simulink model "Astrobee_Simulink_template"  (R2023b)
settings: Solver=FixedStepDiscrete  StartTime=0.0  StopTime=Inf  FixedStep=0.02  RelTol=1e-3  EnableMultiTasking=on
undefined symbols (not defined in the file or in its folder): Header, Wrench
libraries: robotlib x6, simulink x4
settings Model: Creator=The MathWorks, Inc.  LastModifiedBy=Yazan
settings SolverCC: AlgebraicLoopSolver=TrustRegion
settings DataIOCC: LimitDataPoints=on  SaveFormat=Array  ReturnWorkspaceOutputs=off
settings OptimizationCC: ZeroExternalMemoryAtStartup=off  ZeroInternalMemoryAtStartup=off  LifeSpan=Inf  MaxStackSize=64
settings DebuggingCC: SolverPrmCheckMsg=warning  UnconnectedInputMsg=warning  UnconnectedOutputMsg=warning  UnconnectedLineMsg=warning  AllowSymbolicDim=off  SFUnexpectedBacktrackingDiag=warning  SFNoUnconditionalDefaultTransitionDiag=warning  SFExecutionAtInitializationDiag=none  ArithmeticOperatorsInVariantConditions=warning
settings HardwareCC: ProdBitPerPointer=32  ProdBitPerSizeT=32  ProdBitPerPtrDiffT=32  ProdLargestAtomicFloat=None  ProdIntDivRoundTo=Undefined  ProdEndianess=Unspecified  ProdWordSize=32  ProdHWDeviceType=Generic->Unspecified (assume 32-bit Generic)  TargetHWDeviceType=Generic->Unspecified (assume 32-bit Generic)  UseEmbeddedCoderFeatures=off
settings ModelReferenceCC: EnableRefExpFcnMdlSchedulingChecks=on  PropagateSignalLabelsOutOfModel=off
settings SFSimCC: SimUseLocalCustomCode=off  CustomCodeUndefinedFunction=UseInterfaceOnly  SimTargetLang=C++
settings RTWCC: Description=Embedded Coder  SystemTargetFile=ert.tlc  HardwareBoard=Robot Operating System (ROS)  TemplateMakefile=ert_default_tmf  RTWUseLocalCustomCode=off  Toolchain=Catkin  TargetLang=C++
settings CodeAppCC: StateflowObjectComments=on
settings ERTTargetCC: MultiwordLength=2048  ERTCustomFileBanners=off  CodeInterfacePackaging=C++ class  SupportContinuousTime=on  SupportNonInlinedSFcns=on  RemoveResetFunc=off  SupportVariableSizeSignals=on  ModelStepFunctionPrototypeControlCompliant=off  RootIOFormat=Structure reference  ConvertIfToSwitch=off  SuppressUnreachableDefaultCases=off
settings ConfigComp: CovMetricSettings=dw  CovSaveCumulativeToWorkspaceVar=on  CovSaveSingleToWorkspaceVar=on  CovExternalEMLEnable=off  CovSFcnEnable=off

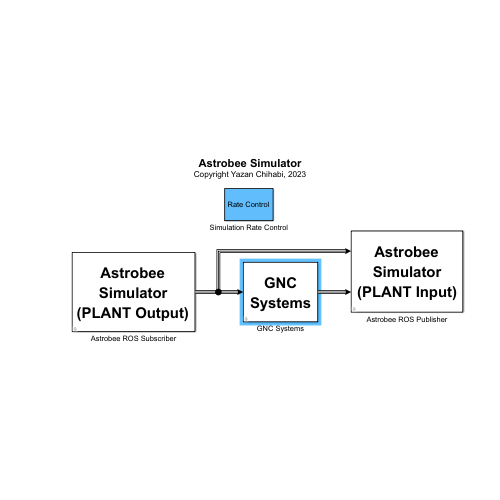
[thumbnail: Simulink's stored preview of the top-level diagram]
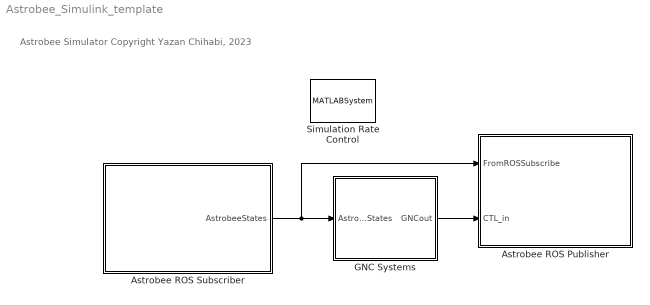
== system Astrobee_Simulink_template ==
  note: Astrobee Simulator
      | Copyright Yazan Chihabi, 2023
  Astrobee ROS Publisher : Subsystem
      mask Display: disp(['{\bf\fontsize{20}Astrobee}' newline newline '{\bf\fontsize{20}Simulator}' newline newline '{\bf\fontsize{20}(PLANT Input)}'], 'texmode','on');
  Astrobee ROS Subscriber : Subsystem
      mask Display: disp(['{\bf\fontsize{20}Astrobee}' newline newline '{\bf\fontsize{20}Simulator}' newline newline '{\bf\fontsize{20}(PLANT Output)}'], 'texmode','on');
  GNC Systems : Subsystem
      mask Display: disp(['{\bf\fontsize{20}GNC}' newline newline '{\bf\fontsize{20}Systems}'], 'texmode','on');
  Simulation Rate Control : MATLABSystem  System=AstrobeeSimulationRateControl  SampleTime=0.02
      mask Type: AstrobeeSimulationRateControl
      mask Display: disp('Rate Control');
  wires:
  Astrobee ROS Subscriber/1(AstrobeeStates) -> Astrobee ROS Publisher/1(FromROSSubscribe), GNC Systems/1(AstrobeeStates)
  GNC Systems/1(GNCout) -> Astrobee ROS Publisher/2(CTL_in)

== system Astrobee_Simulink_template/Astrobee ROS Publisher ==
  FromROSSubscribe : Inport
  CTL_in : Inport  Port=2
  Bus Selector : BusSelector  OutputSignals=HoneyStates.IsNew,BumbleStates.IsNew
  Command Thrust/Torque Publisher (Bumble) : Subsystem
  Command Thrust/Torque Publisher (Honey) : Subsystem
  wires:
  CTL_in/1 -> Command Thrust/Torque Publisher (Honey)/1(CTL_in), Command Thrust/Torque Publisher (Bumble)/1(CTL_in)
  Bus Selector/1 -> Command Thrust/Torque Publisher (Honey)/Enable  "<IsNew>"
  FromROSSubscribe/1 -> Bus Selector/1
  Bus Selector/2 -> Command Thrust/Torque Publisher (Bumble)/Enable  "<IsNew>"

== system Astrobee_Simulink_template/Astrobee ROS Subscriber ==
  Bus Creator : BusCreator  Inputs=2
  ROS Subscriber - Bumble : Subsystem
  ROS Subscriber - Honey : Subsystem
  AstrobeeStates : Outport
  wires:
  ROS Subscriber - Bumble/1(BumbleStates) -> Bus Creator/2
  ROS Subscriber - Honey/1(HoneyStates) -> Bus Creator/1
  Bus Creator/1 -> AstrobeeStates/1

== system Astrobee_Simulink_template/GNC Systems ==
  AstrobeeStates : Inport
  Bumble : Subsystem
      mask Display: disp(['{\bf\fontsize{20}Bumble}' newline newline '{\bf\fontsize{20}GNC}'], 'texmode','on');
  Bus Creator : BusCreator  Inputs=2
  Honey : Subsystem
      mask Display: disp(['{\bf\fontsize{20}Honey}' newline newline '{\bf\fontsize{20}GNC}'], 'texmode','on');
  GNCout : Outport
  wires:
  AstrobeeStates/1 -> Bumble/1(AstrobeeStates), Honey/1(AstrobeeStates)
  Bumble/1(Out1) -> Bus Creator/2
  Honey/1(Out1) -> Bus Creator/1
  Bus Creator/1 -> GNCout/1  "GNCout"

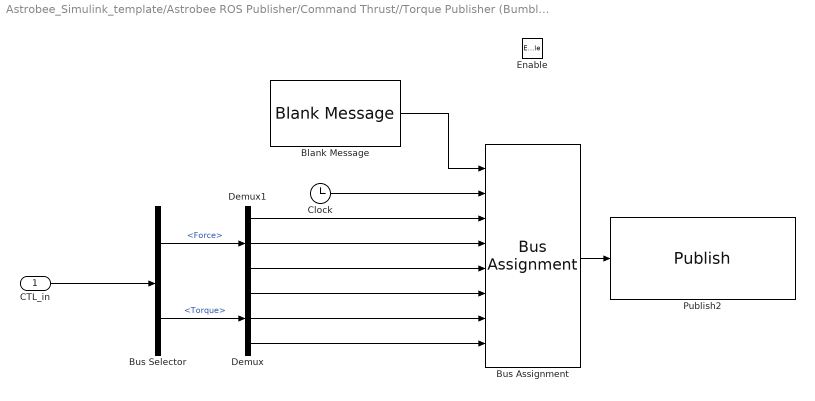
== system Astrobee_Simulink_template/Astrobee ROS Publisher/Command Thrust//Torque Publisher (Bumble) ==
  CTL_in : Inport
  Enable : EnablePort
  Blank Message : robotlib/Blank Message  messageClass=Message  entityType=ff_msgs/FamCommand  messageType=ff_msgs/FamCommand  SampleTime=inf  legacyBusStruct=off
  Bus Assignment : BusAssignment  AssignedSignals=Header.Stamp.Sec,Wrench.Force.X,Wrench.Force.Y,Wrench.Force.Z,Wrench.Torque.X,Wrench.Torque.Y,Wrench.Torque.Z
  Bus Selector : BusSelector  OutputSignals=BumbleCTL.Force,BumbleCTL.Torque
  Clock : Clock
  Demux : Demux  Outputs=3
  Demux1 : Demux  Outputs=3
  Publish2 : robotlib/Publish  topicSource=Select from ROS network  topic=/bumble/gnc/ctl/command  messageType=ff_msgs/FamCommand  legacyBusStruct=off  messageQueueLength=105
  wires:
  CTL_in/1 -> Bus Selector/1
  Bus Selector/1 -> Demux1/1  "<Force>"
  Bus Selector/2 -> Demux/1  "<Torque>"
  Demux1/1 -> Bus Assignment/3
  Demux1/2 -> Bus Assignment/4
  Demux1/3 -> Bus Assignment/5
  Demux/3 -> Bus Assignment/8
  Demux/2 -> Bus Assignment/7
  Demux/1 -> Bus Assignment/6
  Clock/1 -> Bus Assignment/2
  Bus Assignment/1 -> Publish2/1
  Blank Message/1 -> Bus Assignment/1

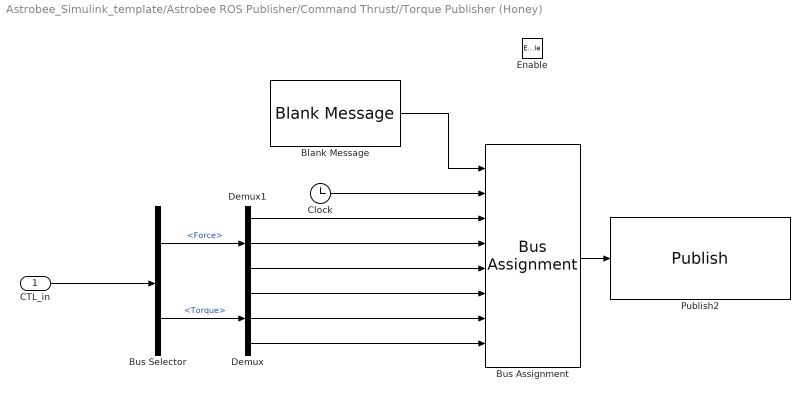
== system Astrobee_Simulink_template/Astrobee ROS Publisher/Command Thrust//Torque Publisher (Honey) ==
  CTL_in : Inport
  Enable : EnablePort
  Blank Message : robotlib/Blank Message  messageClass=Message  entityType=ff_msgs/FamCommand  messageType=ff_msgs/FamCommand  SampleTime=inf  legacyBusStruct=off
  Bus Assignment : BusAssignment  AssignedSignals=Header.Stamp.Sec,Wrench.Force.X,Wrench.Force.Y,Wrench.Force.Z,Wrench.Torque.X,Wrench.Torque.Y,Wrench.Torque.Z
  Bus Selector : BusSelector  OutputSignals=HoneyCTL.Force,HoneyCTL.Torque
  Clock : Clock
  Demux : Demux  Outputs=3
  Demux1 : Demux  Outputs=3
  Publish2 : robotlib/Publish  topicSource=Select from ROS network  topic=/honey/gnc/ctl/command  messageType=ff_msgs/FamCommand  legacyBusStruct=off  messageQueueLength=105
  wires:
  Blank Message/1 -> Bus Assignment/1
  Bus Assignment/1 -> Publish2/1
  Clock/1 -> Bus Assignment/2
  Demux/1 -> Bus Assignment/6
  Demux/2 -> Bus Assignment/7
  Demux/3 -> Bus Assignment/8
  Demux1/3 -> Bus Assignment/5
  Demux1/2 -> Bus Assignment/4
  Demux1/1 -> Bus Assignment/3
  Bus Selector/2 -> Demux/1  "<Torque>"
  Bus Selector/1 -> Demux1/1  "<Force>"
  CTL_in/1 -> Bus Selector/1

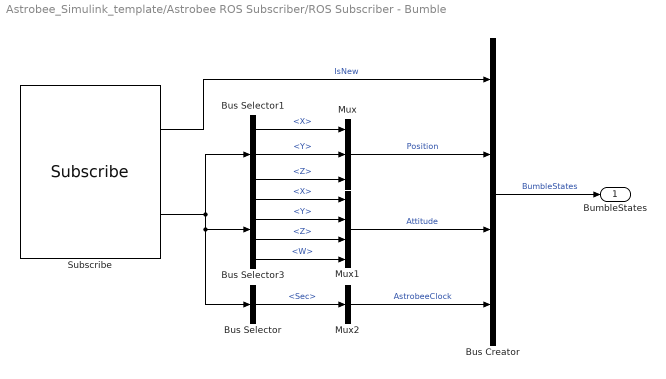
== system Astrobee_Simulink_template/Astrobee ROS Subscriber/ROS Subscriber - Bumble ==
  Bus Creator : BusCreator  Inputs=4
  Bus Selector : BusSelector  OutputSignals=Header.Stamp.Sec
  Bus Selector1 : BusSelector  OutputSignals=Pose.Position.X,Pose.Position.Y,Pose.Position.Z
  Bus Selector3 : BusSelector  OutputSignals=Pose.Orientation.X,Pose.Orientation.Y,Pose.Orientation.Z,Pose.Orientation.W
  Mux : Mux  Inputs=3
  Mux1 : Mux
  Mux2 : Mux  Inputs=1
  Subscribe : robotlib/Subscribe  topicSource=Select from ROS network  topic=/bumble/gnc/ekf  messageType=ff_msgs/EkfState  SampleTime=-1  legacyBusStruct=off  messageQueueLength=51
  BumbleStates : Outport
  wires:
  Bus Creator/1 -> BumbleStates/1  "BumbleStates"
  Bus Selector/1 -> Mux2/1  "<Sec>"
  Bus Selector1/1 -> Mux/1  "<X>"
  Bus Selector1/3 -> Mux/3  "<Z>"
  Bus Selector1/2 -> Mux/2  "<Y>"
  Mux2/1 -> Bus Creator/4  "AstrobeeClock"
  Mux1/1 -> Bus Creator/3  "Attitude"
  Bus Selector3/2 -> Mux1/2  "<Y>"
  Mux/1 -> Bus Creator/2  "Position"
  Bus Selector3/1 -> Mux1/1  "<X>"
  Bus Selector3/3 -> Mux1/3  "<Z>"
  Subscribe/1 -> Bus Creator/1  "IsNew"
  Bus Selector3/4 -> Mux1/4  "<W>"
  Subscribe/2 -> Bus Selector/1, Bus Selector3/1, Bus Selector1/1

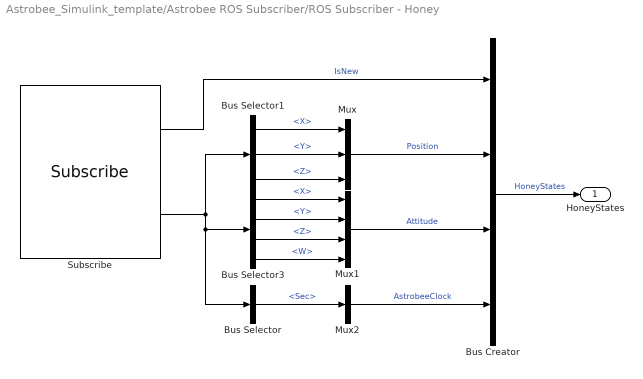
== system Astrobee_Simulink_template/Astrobee ROS Subscriber/ROS Subscriber - Honey ==
  Bus Creator : BusCreator  Inputs=4
  Bus Selector : BusSelector  OutputSignals=Header.Stamp.Sec
  Bus Selector1 : BusSelector  OutputSignals=Pose.Position.X,Pose.Position.Y,Pose.Position.Z
  Bus Selector3 : BusSelector  OutputSignals=Pose.Orientation.X,Pose.Orientation.Y,Pose.Orientation.Z,Pose.Orientation.W
  Mux : Mux  Inputs=3
  Mux1 : Mux
  Mux2 : Mux  Inputs=1
  Subscribe : robotlib/Subscribe  topicSource=Select from ROS network  topic=/honey/gnc/ekf  messageType=ff_msgs/EkfState  SampleTime=-1  legacyBusStruct=off  messageQueueLength=51
  HoneyStates : Outport
  wires:
  Subscribe/2 -> Bus Selector1/1, Bus Selector3/1, Bus Selector/1
  Bus Selector3/4 -> Mux1/4  "<W>"
  Subscribe/1 -> Bus Creator/1  "IsNew"
  Bus Selector3/3 -> Mux1/3  "<Z>"
  Bus Selector3/1 -> Mux1/1  "<X>"
  Mux/1 -> Bus Creator/2  "Position"
  Bus Selector3/2 -> Mux1/2  "<Y>"
  Mux1/1 -> Bus Creator/3  "Attitude"
  Mux2/1 -> Bus Creator/4  "AstrobeeClock"
  Bus Selector1/2 -> Mux/2  "<Y>"
  Bus Selector1/3 -> Mux/3  "<Z>"
  Bus Selector1/1 -> Mux/1  "<X>"
  Bus Selector/1 -> Mux2/1  "<Sec>"
  Bus Creator/1 -> HoneyStates/1  "HoneyStates"

== system Astrobee_Simulink_template/GNC Systems/Bumble ==
  AstrobeeStates : Inport
  Bus Selector : BusSelector  OutputSignals=BumbleStates.IsNew
  Simple Controller : Subsystem
  Out1 : Outport
  wires:
  Simple Controller/1(CTL_out) -> Out1/1  "BumbleCTL"
  AstrobeeStates/1 -> Simple Controller/1(States), Bus Selector/1
  Bus Selector/1 -> Simple Controller/Enable  "<IsNew>"

== system Astrobee_Simulink_template/GNC Systems/Honey ==
  AstrobeeStates : Inport
  Bus Selector : BusSelector  OutputSignals=HoneyStates.IsNew
  Simple Controller : Subsystem
  Out1 : Outport
  wires:
  Bus Selector/1 -> Simple Controller/Enable  "<IsNew>"
  AstrobeeStates/1 -> Bus Selector/1, Simple Controller/1(States)
  Simple Controller/1(CTL_out) -> Out1/1  "HoneyCTL"

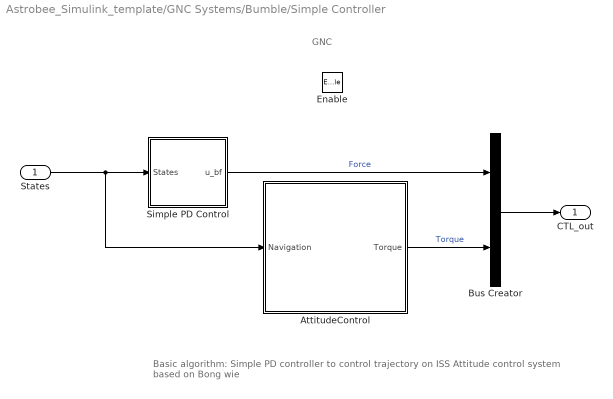
== system Astrobee_Simulink_template/GNC Systems/Bumble/Simple Controller ==
  note: Basic algorithm:
      | Simple PD controller to control trajectory on ISS
      | Attitude control system based on Bong wie
  note: GNC
  States : Inport
  Enable : EnablePort
  AttitudeControl : Subsystem
      mask Display: disp(['{\bf\fontsize{20}Attitude}' newline newline '{\bf\fontsize{20}Control}' newline newline '{\bf\fontsize{20}System}'], 'texmode','on');
  Bus Creator : BusCreator  Inputs=2
  Simple PD Control : Subsystem
  CTL_out : Outport
  wires:
  Bus Creator/1 -> CTL_out/1
  Simple PD Control/1(u_bf) -> Bus Creator/1  "Force"
  AttitudeControl/1(Torque) -> Bus Creator/2  "Torque"
  States/1 -> Simple PD Control/1(States), AttitudeControl/1(Navigation)

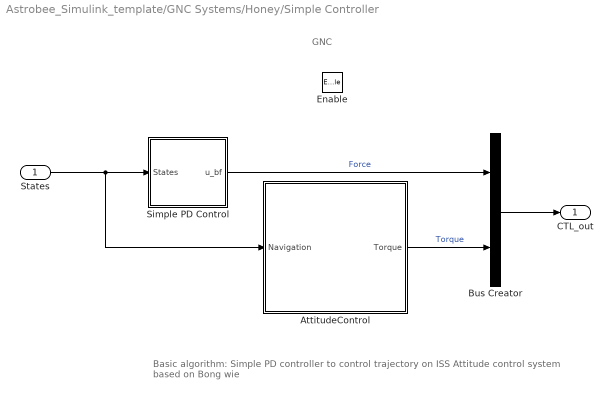
== system Astrobee_Simulink_template/GNC Systems/Honey/Simple Controller ==
  note: GNC
  note: Basic algorithm:
      | Simple PD controller to control trajectory on ISS
      | Attitude control system based on Bong wie
  States : Inport
  Enable : EnablePort
  AttitudeControl : Subsystem
      mask Display: disp(['{\bf\fontsize{20}Attitude}' newline newline '{\bf\fontsize{20}Control}' newline newline '{\bf\fontsize{20}System}'], 'texmode','on');
  Bus Creator : BusCreator  Inputs=2
  Simple PD Control : Subsystem
  CTL_out : Outport
  wires:
  States/1 -> AttitudeControl/1(Navigation), Simple PD Control/1(States)
  AttitudeControl/1(Torque) -> Bus Creator/2  "Torque"
  Simple PD Control/1(u_bf) -> Bus Creator/1  "Force"
  Bus Creator/1 -> CTL_out/1

== system Astrobee_Simulink_template/GNC Systems/Bumble/Simple Controller/AttitudeControl ==
  Navigation : Inport
  AttitudeController : Subsystem
  Constant : Constant  Value=[0;0;0;1]
  QuaternionError : Subsystem
  Torque : Outport  VectorParamsAs1DForOutWhenUnconnected=off
  wires:
  AttitudeController/1(Control) -> Torque/1
  QuaternionError/1(q_error) -> AttitudeController/1(Error)
  Constant/1 -> QuaternionError/1(qd)
  Navigation/1 -> AttitudeController/2(Nav), QuaternionError/2(" Navigation")

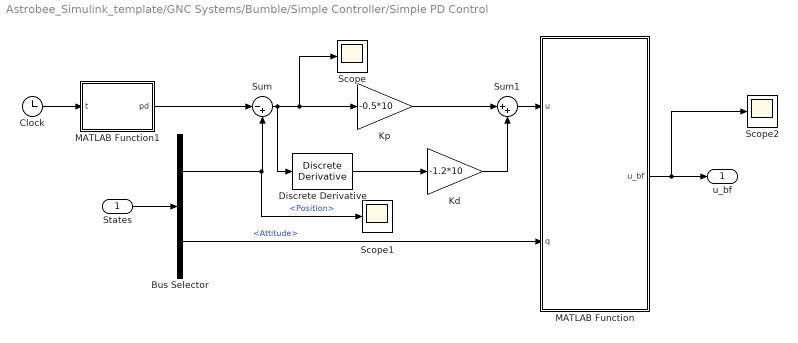
== system Astrobee_Simulink_template/GNC Systems/Bumble/Simple Controller/Simple PD Control ==
  States : Inport
  Bus Selector : BusSelector  OutputSignals=BumbleStates.Position,BumbleStates.Attitude
  Clock : Clock
  Discrete Derivative : simulink/Discrete/Discrete Derivative  gainval=1.0  ICPrevScaledInput=0.0  OutMin=[]  OutMax=[]  OutDataType=fixdt(1, 16)  OutScaling=2^-10  DoSatur=off
  Kd : Gain  Gain=-1.2*10
  Kp : Gain  Gain=-0.5*10
  MATLAB Function : MATLAB Function  TreatAsAtomicUnit=on
  MATLAB Function1 : MATLAB Function  TreatAsAtomicUnit=on
  Scope : Scope
  Scope1 : Scope
  Scope2 : Scope
  Sum : Sum  Inputs=|-+
  Sum1 : Sum  Inputs=|++
  u_bf : Outport
  wires:
  Clock/1 -> MATLAB Function1/1(t)
  Kd/1 -> Sum1/2
  Sum1/1 -> MATLAB Function/1(u)
  MATLAB Function/1(u_bf) -> u_bf/1, Scope2/1
  Bus Selector/2 -> MATLAB Function/2(q)  "<Attitude>"
  Bus Selector/1 -> Sum/2, Scope1/1  "<Position>"
  Kp/1 -> Sum1/1
  States/1 -> Bus Selector/1
  Sum/1 -> Kp/1, Scope/1, Discrete Derivative/1
  MATLAB Function1/1(pd) -> Sum/1
  Discrete Derivative/1 -> Kd/1

== system Astrobee_Simulink_template/GNC Systems/Honey/Simple Controller/AttitudeControl ==
  Navigation : Inport
  AttitudeController : Subsystem
  Constant : Constant  Value=[0;0;sin(-pi/4);cos(-pi/4)]
  QuaternionError : Subsystem
  Torque : Outport  VectorParamsAs1DForOutWhenUnconnected=off
  wires:
  Navigation/1 -> QuaternionError/2(" Navigation"), AttitudeController/2(Nav)
  Constant/1 -> QuaternionError/1(qd)
  QuaternionError/1(q_error) -> AttitudeController/1(Error)
  AttitudeController/1(Control) -> Torque/1

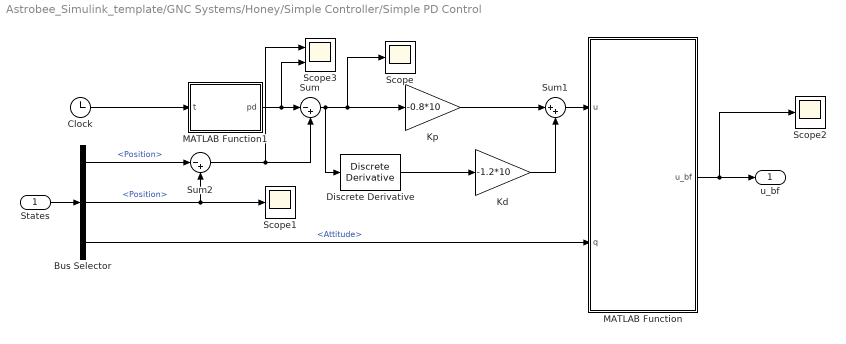
== system Astrobee_Simulink_template/GNC Systems/Honey/Simple Controller/Simple PD Control ==
  States : Inport
  Bus Selector : BusSelector  OutputSignals=BumbleStates.Position,HoneyStates.Position,HoneyStates.Attitude
  Clock : Clock
  Discrete Derivative : simulink/Discrete/Discrete Derivative  gainval=1.0  ICPrevScaledInput=0.0  OutMin=[]  OutMax=[]  OutDataType=fixdt(1, 16)  OutScaling=2^-10  DoSatur=off
  Kd : Gain  Gain=-1.2*10
  Kp : Gain  Gain=-0.8*10
  MATLAB Function : MATLAB Function  TreatAsAtomicUnit=on
  MATLAB Function1 : MATLAB Function  TreatAsAtomicUnit=on
  Scope : Scope
  Scope1 : Scope
  Scope2 : Scope
  Scope3 : Scope  NumInputPorts=2
  Sum : Sum  Inputs=|-+
  Sum1 : Sum  Inputs=|++
  Sum2 : Sum  Inputs=|-+
  u_bf : Outport
  wires:
  Discrete Derivative/1 -> Kd/1
  MATLAB Function1/1(pd) -> Scope3/2, Sum/1
  Sum/1 -> Discrete Derivative/1, Scope/1, Kp/1
  States/1 -> Bus Selector/1
  Kp/1 -> Sum1/1
  Bus Selector/2 -> Scope1/1, Sum2/2  "<Position>"
  Bus Selector/3 -> MATLAB Function/2(q)  "<Attitude>"
  MATLAB Function/1(u_bf) -> Scope2/1, u_bf/1
  Sum1/1 -> MATLAB Function/1(u)
  Kd/1 -> Sum1/2
  Clock/1 -> MATLAB Function1/1(t)
  Bus Selector/1 -> Sum2/1  "<Position>"
  Sum2/1 -> Scope3/1, Sum/2

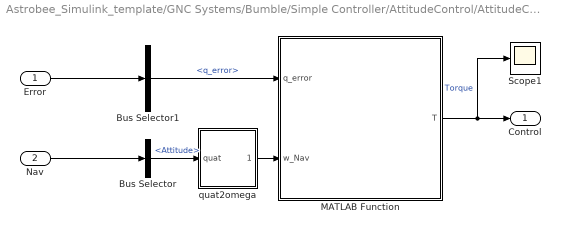
== system Astrobee_Simulink_template/GNC Systems/Bumble/Simple Controller/AttitudeControl/AttitudeController ==
  Error : Inport
  Nav : Inport  Port=2
  Bus Selector : BusSelector  OutputSignals=BumbleStates.Attitude
  Bus Selector1 : BusSelector  OutputSignals=q_error
  MATLAB Function : MATLAB Function  TreatAsAtomicUnit=on
  Scope1 : Scope
  quat2omega : Subsystem
  Control : Outport
  wires:
  Nav/1 -> Bus Selector/1
  Bus Selector/1 -> quat2omega/1(quat)  "<Attitude>"
  quat2omega/1(omega) -> MATLAB Function/2(w_Nav)
  Error/1 -> Bus Selector1/1
  MATLAB Function/1(T) -> Control/1, Scope1/1  "Torque"
  Bus Selector1/1 -> MATLAB Function/1(q_error)  "<q_error>"

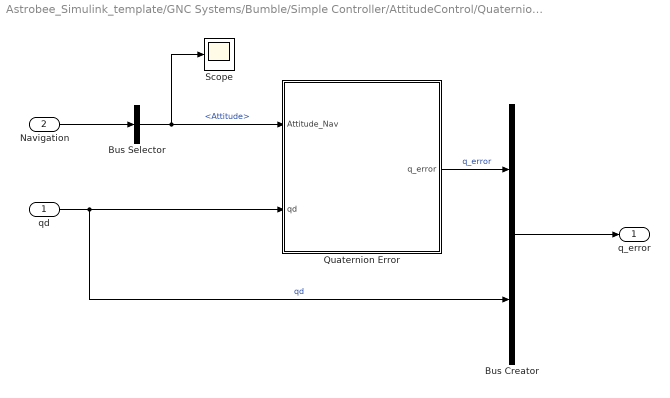
== system Astrobee_Simulink_template/GNC Systems/Bumble/Simple Controller/AttitudeControl/QuaternionError ==
  qd : Inport
  " Navigation" : Inport  Port=2
  Bus Creator : BusCreator  Inputs=2
  Bus Selector : BusSelector  OutputSignals=BumbleStates.Attitude
  Quaternion Error : MATLAB Function  TreatAsAtomicUnit=on
  Scope : Scope
  q_error : Outport  VectorParamsAs1DForOutWhenUnconnected=off
  wires:
  qd/1 -> Quaternion Error/2(qd), Bus Creator/2  "qd"
  Bus Creator/1 -> q_error/1
  Bus Selector/1 -> Scope/1, Quaternion Error/1(Attitude_Nav)  "<Attitude>"
  Quaternion Error/1(q_error) -> Bus Creator/1  "q_error"
  " Navigation"/1 -> Bus Selector/1

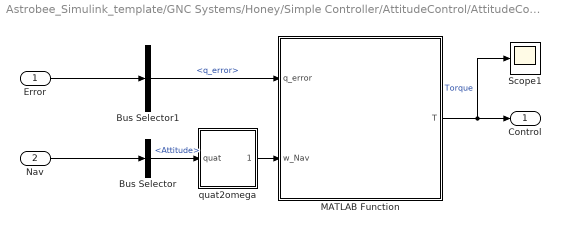
== system Astrobee_Simulink_template/GNC Systems/Honey/Simple Controller/AttitudeControl/AttitudeController ==
  Error : Inport
  Nav : Inport  Port=2
  Bus Selector : BusSelector  OutputSignals=HoneyStates.Attitude
  Bus Selector1 : BusSelector  OutputSignals=q_error
  MATLAB Function : MATLAB Function  TreatAsAtomicUnit=on
  Scope1 : Scope
  quat2omega : Subsystem
  Control : Outport
  wires:
  Bus Selector1/1 -> MATLAB Function/1(q_error)  "<q_error>"
  MATLAB Function/1(T) -> Scope1/1, Control/1  "Torque"
  Error/1 -> Bus Selector1/1
  quat2omega/1(omega) -> MATLAB Function/2(w_Nav)
  Bus Selector/1 -> quat2omega/1(quat)  "<Attitude>"
  Nav/1 -> Bus Selector/1

== system Astrobee_Simulink_template/GNC Systems/Honey/Simple Controller/AttitudeControl/QuaternionError ==
  qd : Inport
  " Navigation" : Inport  Port=2
  Bus Creator : BusCreator  Inputs=2
  Bus Selector : BusSelector  OutputSignals=HoneyStates.Attitude
  Quaternion Error : MATLAB Function  TreatAsAtomicUnit=on
  q_error : Outport  VectorParamsAs1DForOutWhenUnconnected=off
  wires:
  " Navigation"/1 -> Bus Selector/1
  Quaternion Error/1(q_error) -> Bus Creator/1  "q_error"
  Bus Selector/1 -> Quaternion Error/1(Attitude_Nav)  "<Attitude>"
  Bus Creator/1 -> q_error/1
  qd/1 -> Bus Creator/2, Quaternion Error/2(qd)  "qd"

== system Astrobee_Simulink_template/GNC Systems/Bumble/Simple Controller/AttitudeControl/AttitudeController/quat2omega ==
  quat : Inport
  Conversion : MATLAB Function  TreatAsAtomicUnit=on
  Discrete Derivative : simulink/Discrete/Discrete Derivative  gainval=1.0  ICPrevScaledInput=0.0  OutMin=[]  OutMax=[]  OutDataType=fixdt(1, 16)  OutScaling=2^-10  DoSatur=off
  MATLAB Function1 : MATLAB Function  TreatAsAtomicUnit=on
  omega : Outport
  wires:
  quat/1 -> Conversion/1(q)
  MATLAB Function1/1(omega) -> omega/1
  Discrete Derivative/1 -> MATLAB Function1/1(Angle_rate)
  Conversion/1(eul) -> Discrete Derivative/1, MATLAB Function1/2(angle)

== system Astrobee_Simulink_template/GNC Systems/Honey/Simple Controller/AttitudeControl/AttitudeController/quat2omega ==
  quat : Inport
  Conversion : MATLAB Function  TreatAsAtomicUnit=on
  Discrete Derivative : simulink/Discrete/Discrete Derivative  gainval=1.0  ICPrevScaledInput=0.0  OutMin=[]  OutMax=[]  OutDataType=fixdt(1, 16)  OutScaling=2^-10  DoSatur=off
  MATLAB Function1 : MATLAB Function  TreatAsAtomicUnit=on
  omega : Outport
  wires:
  Conversion/1(eul) -> MATLAB Function1/2(angle), Discrete Derivative/1
  Discrete Derivative/1 -> MATLAB Function1/1(Angle_rate)
  MATLAB Function1/1(omega) -> omega/1
  quat/1 -> Conversion/1(q)

== matlab function Astrobee_Simulink_template/GNC Systems/Honey/Simple Controller/AttitudeControl/AttitudeController/MATLAB Function ==
  data: q_error input; T output; w_Nav input
function T  = AttitudeController(q_error,w_Nav)

inertiaMatrix = [0.1422,0,0;
    0,0.1422,0;
    0,0,0.1422];
%% ATTITUDE CONTROL %%
%{   
    Run a quaternion-based PD-like attitude controller that minimizes
    the axis error. If q1_error, q2_error, and q3_error are zero, then
    q4_error must be 1 and therefore there is zero error. So, we must
    drive q1_error, q2_error, and q3_error to zero. The sign of 
    q4_error is used to guide the direction.
    
    Controller adapted from: https://arc.aiaa.org/doi/abs/10.2514/3.19988?journalCode=jgcd
    Dr. Bong Wie Attitude Controller
    Inputs: 
        - quaternion_error_in_servicer_body_frame (4 components, the first 3 are the axis components and the 4th is the angle component)
        - angular_rate_error_in_servicer_body_frame (3 angular rate errors in rad/s in the body-fixed reference frame)
%}

% T = (sign(q_error(4))+(q_error(4) == 0))*Kp_Attitude*q_error(1:3) + Kd_Attitude*w_error;

% T = [0;0;0];
%% Different version of Dr. Bong Wie Attitude Controller
%{   
    Quarternion feedback regulator for spacecraft eigenaxis rotations
    B. Wie, H. Weiss and A. Arapostathis https://doi.org/10.2514/3.20418
%}
    q=q_error(1:3); %error quaternions
    T = (-6*inertiaMatrix*q)+(-12*inertiaMatrix*w_Nav)-(cross(w_Nav,inertiaMatrix*(w_Nav)));
end

== matlab function Astrobee_Simulink_template/GNC Systems/Honey/Simple Controller/AttitudeControl/AttitudeController/quat2omega/Conversion ==
  data: eul output; q input
function eul = quat2eul(q)
%#codegen

% Convert the quaternion to euler angles

C = quat2rot(q);

roll = atan2(C(2,3),C(3,3));
pitch = -asin(C(1,3));
yaw = atan2(C(1,2),C(1,1));

eul = [roll;pitch;yaw];
end

== matlab function Astrobee_Simulink_template/GNC Systems/Honey/Simple Controller/AttitudeControl/QuaternionError/Quaternion Error ==
  data: Attitude_Nav input; q_error output size=4; qd input
function q_error  = q_err_calc(Attitude_Nav,qd)


%% Quaternion Error
q_Nav = Attitude_Nav(1:4);
q_Nav = NormalizeQuaternion(q_Nav);

qm = [ qd(4), qd(3),-qd(2),-qd(1);
      -qd(3), qd(4), qd(1),-qd(2);
       qd(2),-qd(1), qd(4),-qd(3);
       qd(1), qd(2), qd(3), qd(4)];
   
q_error = (qm * q_Nav);

q_error = NormalizeQuaternion(q_error); % normalizing and ensuring q(4) is positive

if isnan(q_error)
    q_error = [0;0;0;0];
end


end

== matlab function Astrobee_Simulink_template/GNC Systems/Bumble/Simple Controller/AttitudeControl/AttitudeController/MATLAB Function ==
  data: q_error input; T output; w_Nav input
function T  = AttitudeController(q_error,w_Nav)

inertiaMatrix = [0.1422,0,0;
    0,0.1422,0;
    0,0,0.1422];
%% ATTITUDE CONTROL %%
%{   
    Run a quaternion-based PD-like attitude controller that minimizes
    the axis error. If q1_error, q2_error, and q3_error are zero, then
    q4_error must be 1 and therefore there is zero error. So, we must
    drive q1_error, q2_error, and q3_error to zero. The sign of 
    q4_error is used to guide the direction.
    
    Controller adapted from: https://arc.aiaa.org/doi/abs/10.2514/3.19988?journalCode=jgcd
    Dr. Bong Wie Attitude Controller
    Inputs: 
        - quaternion_error_in_servicer_body_frame (4 components, the first 3 are the axis components and the 4th is the angle component)
        - angular_rate_error_in_servicer_body_frame (3 angular rate errors in rad/s in the body-fixed reference frame)
%}

% T = (sign(q_error(4))+(q_error(4) == 0))*Kp_Attitude*q_error(1:3) + Kd_Attitude*w_error;

% T = [0;0;0];
%% Different version of Dr. Bong Wie Attitude Controller
%{   
    Quarternion feedback regulator for spacecraft eigenaxis rotations
    B. Wie, H. Weiss and A. Arapostathis https://doi.org/10.2514/3.20418
%}
    q=q_error(1:3); %error quaternions
    T = (-6*inertiaMatrix*q)+(-12*inertiaMatrix*w_Nav)-(cross(w_Nav,inertiaMatrix*(w_Nav)));
end

== matlab function Astrobee_Simulink_template/GNC Systems/Bumble/Simple Controller/AttitudeControl/AttitudeController/quat2omega/Conversion ==
  data: eul output; q input
function eul = quat2eul(q)
%#codegen

% Convert the quaternion to euler angles

C = quat2rot(q);

roll = atan2(C(2,3),C(3,3));
pitch = -asin(C(1,3));
yaw = atan2(C(1,2),C(1,1));

eul = [roll;pitch;yaw];
end

== matlab function Astrobee_Simulink_template/GNC Systems/Honey/Simple Controller/AttitudeControl/AttitudeController/quat2omega/MATLAB Function1 ==
  data: Angle_rate input; omega output; angle input
function omega = EulerRates2Omega(Angle_rate,angle)

roll = angle(1);
roll_dot = Angle_rate(1);
pitch = angle(2);
pitch_dot = Angle_rate(2);
yaw = angle(3);
yaw_dot = Angle_rate(3);

Phi = [1 0 -sin(pitch);
    0 cos(roll) -sin(roll);
    0 sin(roll)/cos(pitch) cos(roll)/cos(pitch)];

omega = Phi*[roll_dot;pitch_dot;yaw_dot];

end

== matlab function Astrobee_Simulink_template/GNC Systems/Bumble/Simple Controller/AttitudeControl/AttitudeController/quat2omega/MATLAB Function1 ==
  data: Angle_rate input; omega output; angle input
function omega = EulerRates2Omega(Angle_rate,angle)

roll = angle(1);
roll_dot = Angle_rate(1);
pitch = angle(2);
pitch_dot = Angle_rate(2);
yaw = angle(3);
yaw_dot = Angle_rate(3);

Phi = [1 0 -sin(pitch);
    0 cos(roll) -sin(roll);
    0 sin(roll)/cos(pitch) cos(roll)/cos(pitch)];

omega = Phi*[roll_dot;pitch_dot;yaw_dot];

end

== matlab function Astrobee_Simulink_template/GNC Systems/Bumble/Simple Controller/AttitudeControl/QuaternionError/Quaternion Error ==
  data: Attitude_Nav input; q_error output size=4; qd input
function q_error  = q_err_calc(Attitude_Nav,qd)


%% Quaternion Error
q_Nav = Attitude_Nav(1:4);
q_Nav = NormalizeQuaternion(q_Nav);

qm = [ qd(4), qd(3),-qd(2),-qd(1);
      -qd(3), qd(4), qd(1),-qd(2);
       qd(2),-qd(1), qd(4),-qd(3);
       qd(1), qd(2), qd(3), qd(4)];
   
q_error = (qm * q_Nav);

q_error = NormalizeQuaternion(q_error); % normalizing and ensuring q(4) is positive

if isnan(q_error)
    q_error = [0;0;0;0];
end


end

== matlab function Astrobee_Simulink_template/GNC Systems/Honey/Simple Controller/Simple PD Control/MATLAB Function ==
  data: u input; u_bf output; q input
function u_bf = Rotate2Body(u,q)

C = quat2rot(q);

u_bf = C*u;

end

== matlab function Astrobee_Simulink_template/GNC Systems/Honey/Simple Controller/Simple PD Control/MATLAB Function1 ==
  data: t input; pd output
function pd = fcn(t)

pd = [0;4;0.5];

% pd = [0.5*cos(0.05*t +0.5*pi);0.5*sin(0.05*t +0.5*pi);0];

end

== matlab function Astrobee_Simulink_template/GNC Systems/Bumble/Simple Controller/Simple PD Control/MATLAB Function ==
  data: u input; u_bf output; q input
function u_bf = Rotate2Body(u,q)

C = quat2rot(q);

u_bf = C*u;

end

== matlab function Astrobee_Simulink_template/GNC Systems/Bumble/Simple Controller/Simple PD Control/MATLAB Function1 ==
  data: t input; pd output
function pd = fcn(t)

pd = [11;-8;5];

% pd = [11+(0.5*cos(0.05*t));-6+(0.5*sin(0.05*t));5];

end
